simulink model "CAE_FP2"  (R2023b)
settings: Solver=VariableStepAuto  StartTime=0.0  StopTime=10.0  MaxStep=0.001  RelTol=1e-3
undefined symbols (not defined in the file or in its folder): magnitude
settings Model: Creator=Wojciech Zub  LastModifiedBy=Wojciech Zub

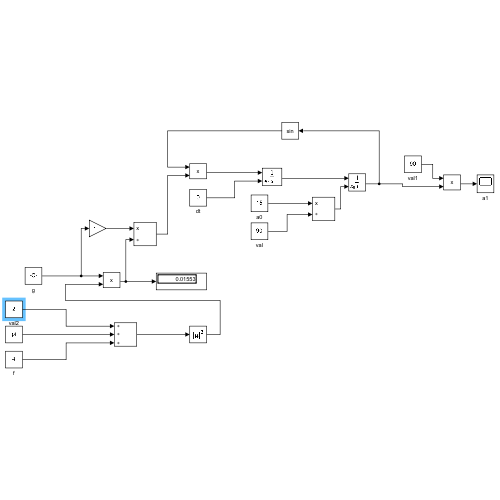
[thumbnail: Simulink's stored preview of the top-level diagram]
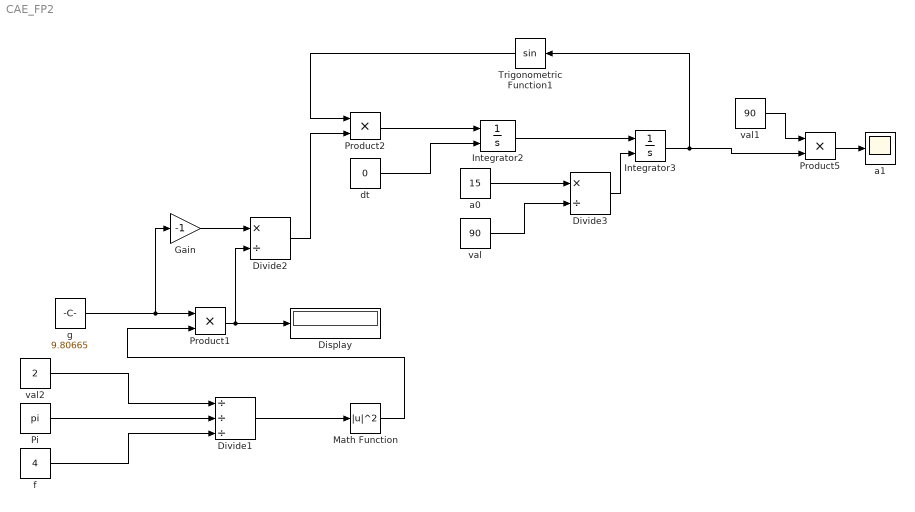
== system CAE_FP2 ==
  Display : Display
  Divide1 : Product  Inputs=///
  Divide2 : Product  Inputs=*/
  Divide3 : Product  Inputs=*/
  Gain : Gain  Gain=-1
  Integrator2 : Integrator  InitialConditionSource=external
  Integrator3 : Integrator  InitialConditionSource=external
  Math Function : Math  Operator=magnitude^2
  Pi : Constant  Value=pi  OutDataTypeStr=Inherit: Inherit via back propagation
  Product1 : Product
  Product2 : Product
  Product5 : Product
  Trigonometric Function1 : Trigonometry
  a0 : Constant  Value=15
  a1 : Scope
  dt : Constant  Value=0
  f : Constant  Value=4
  g : Constant  Value=9.80665
  val : Constant  Value=90
  val1 : Constant  Value=90
  val2 : Constant  Value=2
  wires:
  f/1 -> Divide1/3
  val2/1 -> Divide1/1
  Pi/1 -> Divide1/2
  Divide1/1 -> Math Function/1
  Math Function/1 -> Product1/2
  Product1/1 -> Divide2/2, Display/1
  a0/1 -> Divide3/1
  Product5/1 -> a1/1
  Integrator2/1 -> Integrator3/1
  Trigonometric Function1/1 -> Product2/1
  Integrator3/1 -> Trigonometric Function1/1, Product5/2
  Product2/1 -> Integrator2/1
  Divide2/1 -> Product2/2
  val1/1 -> Product5/1
  Divide3/1 -> Integrator3/2
  val/1 -> Divide3/2
  dt/1 -> Integrator2/2
  g/1 -> Product1/1, Gain/1
  Gain/1 -> Divide2/1
